simulink model "HeartSignals"  (R2017b)
settings: Solver=FixedStepDiscrete  StartTime=0.0  StopTime=inf  FixedStep=1/200  RelTol=1e-3  EnableMultiTasking=on
libraries: tftlibrary x2, arduinolib x1
settings Model: ExtModeTrigDuration=2  Creator=mgovinda  LastModifiedBy=mgovinda
settings OptimizationCC: PassReuseOutputArgsAs=Individual arguments  MaxStackSize=64
settings DebuggingCC: ParameterTunabilityLossMsg=error
settings HardwareCC: ProdBitPerInt=16  ProdBitPerPointer=16  ProdBitPerSizeT=16  ProdBitPerPtrDiffT=16  ProdLargestAtomicFloat=None  ProdWordSize=8  ProdHWDeviceType=Atmel->AVR
settings SFSimCC: MATLABDynamicMemAlloc=off
settings RTWCC: SystemTargetFile=ert.tlc  HardwareBoard=Arduino Uno  TLCOptions=-aInlineSetEventsForThisBaseRateFcn=TLC_FALSE -aSuppressMultiTaskScheduler=TLC_FALSE -aRateBasedStepFcn=1  TemplateMakefile=ert_default_tmf  GenerateReport=on  Toolchain=Arduino AVR  BuildConfiguration=Faster Runs  IncludeHyperlinkInReport=on  GenerateTraceInfo=on  GenerateTraceReport=on  GenerateTraceReportSl=on  GenerateTraceReportSf=on  GenerateTraceReportEml=on
settings CodeAppCC: ForceParamTrailComments=on  IgnoreCustomStorageClasses=off  OperatorAnnotations=on  SimulinkDataObjDesc=on  SFDataObjDesc=on  MATLABFcnDesc=on  InsertBlockDesc=on  StateflowObjectComments=on  MATLABSourceComments=on
settings ERTTargetCC: SupportContinuousTime=on  SupportVariableSizeSignals=on
settings SimscapeCC: SimscapeNormalizeSystem=off

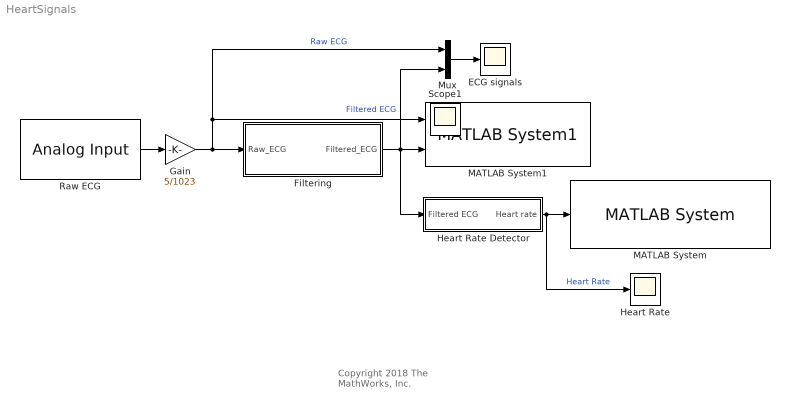
== system HeartSignals ==
  note: Copyright 2018 The MathWorks, Inc.
  ECG signals : Scope
  Filtering : Subsystem
  Gain : Gain  Gain=5/1023  OutDataTypeStr=double
  Heart Rate : Scope
  Heart Rate Detector : Subsystem
  MATLAB System : tftlibrary/MATLAB System  txtColor_=White  txtSize_=uint8( 5 )  x_=0  y_=0
  MATLAB System1 : tftlibrary/MATLAB System1  line1Color_=Green  line2Color_=Red
  Mux : Mux  Inputs=2
  Raw ECG : arduinolib/Analog Input  pinNumber=0  ReadResultsOnly=off  ConversionTriggerSource=Software  ExternalTriggerType=uint32(0)  OutputDataType=uint16  EnableConversionCompleteNotify=off  EnableOuputStatus=off  SampleTime=1/200  blockPlatform=arduino
  Scope1 : Scope
  wires:
  Raw ECG/1 -> Gain/1
  Gain/1 -> Filtering/1(Raw_ECG), MATLAB System1/1, Mux/1  "Raw ECG"
  Filtering/1(Filtered_ECG) -> MATLAB System1/2, Mux/2, Heart Rate Detector/1(Filtered ECG)  "Filtered ECG"
  Heart Rate Detector/1(Heart rate) -> MATLAB System/1, Heart Rate/1  "Heart Rate"
  Mux/1 -> ECG signals/1

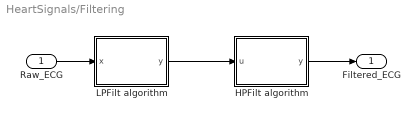
== system HeartSignals/Filtering ==
  Raw_ECG : Inport
  HPFilt algorithm : MATLAB Function  TreatAsAtomicUnit=on
  LPFilt algorithm : MATLAB Function  TreatAsAtomicUnit=on
  Filtered_ECG : Outport
  wires:
  HPFilt algorithm/1(y) -> Filtered_ECG/1
  LPFilt algorithm/1(y) -> HPFilt algorithm/1(u)
  Raw_ECG/1 -> LPFilt algorithm/1(x)

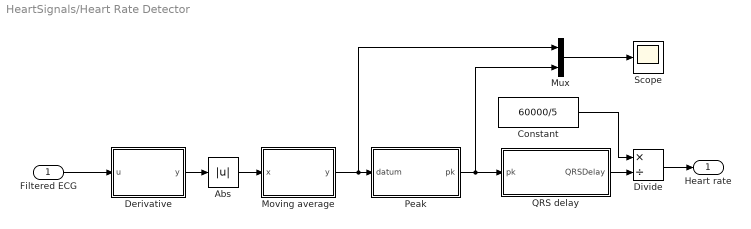
== system HeartSignals/Heart Rate Detector ==
  Filtered ECG : Inport
  Abs : Abs
  Constant : Constant  Value=60000/5  OutDataTypeStr=int16
  Derivative : MATLAB Function  TreatAsAtomicUnit=on
  Divide : Product  Inputs=*/
  Moving average : MATLAB Function  TreatAsAtomicUnit=on
  Mux : Mux  Inputs=2
  Peak : MATLAB Function  TreatAsAtomicUnit=on
  QRS delay : MATLAB Function  TreatAsAtomicUnit=on
  Scope : Scope
  Heart rate : Outport
  wires:
  Abs/1 -> Moving average/1(x)
  Moving average/1(y) -> Mux/1, Peak/1(datum)
  Filtered ECG/1 -> Derivative/1(u)
  Derivative/1(y) -> Abs/1
  Peak/1(pk) -> Mux/2, QRS delay/1(pk)
  QRS delay/1(QRSDelay) -> Divide/2
  Divide/1 -> Heart rate/1
  Constant/1 -> Divide/1
  Mux/1 -> Scope/1

== matlab function HeartSignals/Filtering/HPFilt algorithm ==
  data: u input; y output
function y = hpfilt(u)
    %  hpfilt() implements the high pass filter represented by the following
    %  difference equation:
    %
    %       x[n] = x[n-1] + u[n] - u[n-32]
    %       y[n] = u[n-16] - x[n] ;
    %
    %  Note that the filter delay is 15.5 samples
    
    % Circular buffer n
coder.inline('never');
    persistent x z n
    y = cast(0,'like',u);
    if isempty(x)
        x = zeros(1,1,'like',u);
        z = zeros(32,1,'like',u);
        n = int16(0);
    end
    x(:) = x + u - z(n+1);
    half_n = bitand(n - 16, int16(31));
    
    y = z(half_n+1);
    y(:) = y - bitsra(x,5);
    z(n+1) = u;
    n(:) = bitand(n + 1, int16(31));
end

== matlab function HeartSignals/Filtering/LPFilt algorithm ==
  data: x input; y output
function y = lpfilt(x)
%  lpfilt() implements the digital filter represented by the difference
%  equation:
%
% 	y[n] = 2*y[n-1] - y[n-2] + x[n] - 2*x[n-5] + x[n-10]
%
%	Note that the filter delay is five samples.
%
%  y(n) = 2*y(n-1) - y(n-2) + x(n) - 2*x(n-5) + x(n-10)
%
%       1*y(n) - 2*y(n-1) + 1*y(n-2) = 1*x(n) + 0*x(n-1) + 0*x(n-2) + 0*x(n-3) +  0*x(n-4) - 2*x(n-5) + 0*x(n-6) + 0*x(n-7) + 0*x(n-8)  + 0*x(n-9) + 1*x(n-10)
%  a = [1       -2          1];   b = [1        0          0          0           0         -2          0          0          0           0          1];
%
% Lowpass filter coefficients.  The roots of a are on the unit circle, but
% they exactly cancel with roots of b.
% Dividing numerator and denominator gives q = [1 2 3 4 5 4 3 2 1].
% It's counting on perfect cancellation in order to get a filter that only
% has powers of two for coefficients.
% b = [1  0   0   0    0  -2   0   0   0    0   1];
% a = [1  -2  1];
% roots_a = roots(a)
% [q,r] = deconv(b,a) %#ok<*NOPTS>
coder.inline('never');
    persistent x1 x2 x3 x4 x5 x6 x7 x8 x9 x10
    persistent y1 y2
    y = cast(0,'like',x);
    y0 = cast(0,'like',x);
    if isempty(x1)
        x1 = cast(0,'like',x);
        x2 = cast(0,'like',x);
        x3 = cast(0,'like',x);
        x4 = cast(0,'like',x);
        x5 = cast(0,'like',x);
        x6 = cast(0,'like',x);
        x7 = cast(0,'like',x);
        x8 = cast(0,'like',x);
        x9 = cast(0,'like',x);
        x10 = cast(0,'like',x);
        y1 = cast(0,'like',x);
        y2 = cast(0,'like',x);
    end
    y0(:) = bitsll(y1,1) - y2 + x - bitsll(x5,1) + x10;
    y2(:) = y1;
    y1(:) = y0;

    y(:) = bitsra(y0,5);

    x10 = x9;
    x9  = x8;
    x8  = x7;
    x7  = x6;
    x6  = x5;
    x5  = x4;
    x4  = x3;
    x3  = x2;
    x2  = x1;
    x1  = x;
end

== matlab function HeartSignals/Heart Rate Detector/Derivative ==
  data: u input; y output
function y = deriv1(u)
%  derivative implements the derivative approximation represented by
%  the difference equation:
%
%	y[n] = 2*x[n] + x[n-1] - x[n-3] - 2*x[n-4]
%
%  The filter has a delay of 2.

    coder.inline('never');
    persistent x1 x2 x3 x4
    if isempty(x1)
        x1 = cast(0,'like',u);
        x2 = cast(0,'like',u);
        x3 = cast(0,'like',u);
        x4 = cast(0,'like',u);
    end
    y = cast(0,'like',u);
    y(:) = bitsll(u,1) + x1 - x3 - bitsll(x4,1);
    x4 = x3;
    x3 = x2;
    x2 = x1;
    x1 = u;
 end

== matlab function HeartSignals/Heart Rate Detector/Moving average ==
  data: x input; y output
function y = mvwint(x)
% mvwint() implements a moving window integrator, averaging
% the signal values over the last 16

    persistent runningSum
    persistent x0 x1 x2 x3 x4 x5 x6 x7 x8 x9 x10
    persistent x11 x12 x13 x14 x15
    y = cast(0,'like',x);
    if isempty(runningSum)
        runningSum = cast(0, 'like', x);
        x0 = cast(0, 'like', x);
        x1 = cast(0, 'like', x);
        x2 = cast(0, 'like', x);
        x3 = cast(0, 'like', x);
        x4 = cast(0, 'like', x);
        x5 = cast(0, 'like', x);
        x6 = cast(0, 'like', x);
        x7 = cast(0, 'like', x);
        x8 = cast(0, 'like', x);
        x9 = cast(0, 'like', x);
        x10 = cast(0, 'like', x);
        x11 = cast(0, 'like', x);
        x12 = cast(0, 'like', x);
        x13 = cast(0, 'like', x);
        x14 = cast(0, 'like', x);
        x15 = cast(0, 'like', x);
        return
    end
    
    runningSum(:) = runningSum - x15;
    x15 = x14;
    x14 = x13;
    x13 = x12;
    x12 = x11;
    x11 = x10;
    x10 = x9;
    x9 = x8;
    x8 = x7;
    x7 = x6;
    x6 = x5;
    x5 = x4;
    x4 = x3;
    x3 = x2;
    x2 = x1;
    x1 = x0;
    x0 = x;
    runningSum(:) = runningSum + x0;
    y(:) = bitsra(runningSum,4);
end

== matlab function HeartSignals/Heart Rate Detector/Peak ==
  data: datum input; pk output
function pk = peak(datum)
    % peak() takes a datum as input and returns a peak height
    % when the signal returns to half its peak height, or it has been
    % 95 ms since the peak height was detected.
    
    persistent maxPeak lastDatum timeSinceMax
    pk = cast(0,'like',datum);
    if isempty(maxPeak)
        maxPeak = cast(0,'like',datum);
        lastDatum = cast(0,'like',datum);
        timeSinceMax = uint16(0);
        return
    end
    
    if timeSinceMax > 0
        timeSinceMax(:) = timeSinceMax + 1;
    end
    
    if((datum > lastDatum) && (datum > maxPeak)) % rising slope
        maxPeak(:) = datum ;
        if(maxPeak > 2) % reset timeSinceMax 
            % Not sure what maxPeak > 2 means with scaling?
            timeSinceMax(:) = 1 ;
        end
    elseif(datum < bitsra(maxPeak,1)) % middle of falling slope
        % Less than half the peak height
        pk(:) = maxPeak ;
        maxPeak(:) = 0 ;
        timeSinceMax(:) = 0 ;
    elseif(timeSinceMax > int16(19))
        pk(:) = maxPeak ;
        maxPeak(:) = 0 ;
        timeSinceMax(:) = 0 ;
    end
    lastDatum = datum ;
end

== matlab function HeartSignals/Heart Rate Detector/QRS delay ==
  data: pk input; QRSDelay output
function QRSDelay  = qrs_delay(pk)
    persistent count
    persistent lastQRSDelay
    persistent threshold
    % Normal low range for a QRS detection is 60ms.
    % Characteristics of the Normal ECG. Frank G. Yanowitz,
    % MD. Professor of Medicine. University of Utah School of
    % Medicine. http://ecg.utah.edu.
    qrs_duration_in_samples = int32(60e-3 * 5);
    if isempty(lastQRSDelay)
        count = int16(0);
        lastQRSDelay = int16(0);
        threshold = cast(4, 'like', pk);
    end
    count(:) = count + 1;
    threshold(:) = filter8(pk);
    if pk > threshold && count > qrs_duration_in_samples
        lastQRSDelay(:) = count;
        count(:) = 0;
    end
    QRSDelay = lastQRSDelay;
    thisThreshold = threshold;
end

function y = filter8(x)
    persistent n
    persistent z
    persistent lastY
    if isempty(n)
        n = uint8(0);
        z = zeros(8,1,'like',x);
        lastY = cast(0,'like',x);
    end
    if x ~= cast(0,'like',x)
        z(n+1) = x;
        n = bitand(n+1,uint8(7));
        lastY(:) = sum(bitsra(z,3));
    end
    y = lastY;
end
